simulink model "CML_Iso_Force_Matching"  (R2015a)
settings: Solver=ode4  SolverMode=MultiTasking  StartTime=0.0  StopTime=inf  FixedStep=BKIN_STEP_TIME  RelTol=1e-3
StartFcn:
  |  warndlg('Dexterit-E models cannot run under simulation. Please compile your model and run it from within Dexterit-E.');set_param(bdroot,'SimulationCommand','stop')
model workspace (MAT data in the model file):
  BKIN_STEP_TIME = 0.00025
  col_x = 1
  col_y = 2
  VRAD = 3
  COLOR = 4
  TARGET_COL = 2
  BKIN_KINEMATIC_FRAME_SIZE = 400
  E_NO_EVENT = 0
  INIT_DUR = 5
  TP_ITI = 11
  K_JOINT_ASSESSED = 3
  TEXT1 = 5
  TEXT2 = 6
  HEIGHT = 8
  STROKE_WIDTH = 9
  GOAL_F_PCT = 3
  DO_FDBK = 10
  MAX_MOVE_TIME = 9
  MIN_FORCE = 4
  E_TEST_MVC = 1
  E_HOLD_MVC = 3
  E_EOT = 30
  E_FORCE_TRIAL = 11
  E_HOLD_FORCE = 13
  K_BAR_TGT = 4
  K_MVC_TEXT_TGT = 5
  E_INIT_FORCE = 12
  E_SET_MVC = 2
  TRIAL_TYPE = 1
  TEST_ARM = 8
  E_REST_FORCE = 14
  E_INIT_MATCH_FORCE = 15
  E_HOLD_MATCH_FORCE = 16
  TEXT3 = 7
  K_MVC = 6
  E_ACCEPT_MVC = 5
  ACCEPT_MVC = 2
  REJECT_MVC = 3
  K_ARM1_TGT = 1
  K_ARM2_TGT = 2
  E_FATIGUE_TRIAL = 21
  E_INIT_FATIGUE = 22
  E_HOLD_FATIGUE = 23
  HOLD_TIME = 6
  REST_TIME = 7
  E_CHECK_MVC = 4
  E_REJECT_MVC = 6
  K_SUR_TGT = 7
  K_SUR_TEXT_TGT = 8
  TEXT4 = 10
  AUDIO_FDBK_TYPE = 12
libraries: Video x8, simulink x7, slrtlib x7, General x3, KINARM_loads x3, KINARM_IO x2, KINARM_general x2, xpcnilib x1
(part 2 of 2)

== matlab function CML_Iso_Force_Matching/Subsystem1/Trajectory Arm1/calculate robot scaling/MATLAB Function ==
  data: robot_type input; scaling output; exo_scaling input
function scaling = fcn(robot_type, exo_scaling)
%#codegen

scaling = [0, 0];

%0 = EXO, 1 = EP, 2 = NHP
for n=1:2
    if robot_type(n) == 1
        scaling(n) = 0;
    else
        scaling(n) = exo_scaling(n);
    end
end

== matlab function CML_Iso_Force_Matching/Subsystem1/Trajectory Arm1/Create_Trajectory/Virtual_Trajectory/Extract_Position ==
  settings: fimath=|
      | fimath(...
      | 'RoundMode', 'floor',...
      | 'OverflowMode', 'wrap',...
      | 'ProductMode', 'KeepLSB', 'ProductWordLength', 32,...
      | 'SumMode', 'KeepLSB', 'SumWordLength', 32,...
      | 'CastBeforeSum', false)
  data: u input; position output
function position = fcn(u)

position=[0,0];	%initialization
if length(u)==2	%input is assumed to be (x,y) position, global coordinates, (m)		
	position=u;
else			%input is assumed to be a VCODE
	position(1)=u(3);
	position(2)=u(4);
end

== matlab function CML_Iso_Force_Matching/Subsystem1/Trajectory Arm1/Create_Trajectory/Virtual_Trajectory/Extract_Position1 ==
  settings: fimath=|
      | fimath(...
      | 'RoundMode', 'floor',...
      | 'OverflowMode', 'wrap',...
      | 'ProductMode', 'KeepLSB', 'ProductWordLength', 32,...
      | 'SumMode', 'KeepLSB', 'SumWordLength', 32,...
      | 'CastBeforeSum', false)
  data: u input; position output
function position = fcn(u)

position=[0,0];	%initialization
if length(u)==2	%input is assumed to be (x,y) position, global coordinates, (m)		
	position=u;
else			%input is assumed to be a VCODE
	position(1)=u(3);
	position(2)=u(4);
end

== matlab function CML_Iso_Force_Matching/Force_Fdbk_Bar/MakeBar ==
  data: currforce input; VCODES output; mvc input; goalforce input; VCODE input; heightratio output
function [VCODES,heightratio] = fcn(currforce,mvc,goalforce,VCODE)
%#codegen

%calculate the height ratio to scale the inner bar by
heightratio = currforce/(mvc*goalforce/100); %the top of the bar is always the goal force
if heightratio > 1
    heightratio = 1;
elseif heightratio < 0
    heightratio = 0;
end

%duplicate the rectangle shape; VCODE(2,:) will be the inner fill bar,
% VCODE(1,:) will be the outer border
VCODES = [VCODE; VCODE];

%VCODE(1,:) specifies a fill color and no stroke color; we want to make the
%outline have no fill and a white border
VCODES(2,7) = 0; %remove the stroke width on the inner bar
VCODES(2,10) = VCODES(2,10)*.9; %shrink the width of the inner bar to fill the frame
VCODES(1,5) = createcolor(0,0,0); %set the outer frame fill to black
VCODES(1,6) = createcolor(100,100,100); %set the outer frame stroke to white

%the rectangle has dims (10,11,12) = width (x dir), height (y dir), rot
%we want to scale the inner rect height by the heightratio
VCODES(2,11) = VCODES(2,11)*heightratio;
%we need to edit the y position of the inner bar to keep the base fixed at
%the bottom of the outer frame, by subtracting half the height difference
%between the two bars
VCODES(2,4) = VCODES(2,4) - ( VCODES(1,11) - VCODES(2,11) )/2;  


% 
% %we need to add in a line representing the target height.
% VCODES(3,1) = 4; %set this to be a line segment
% 
% framewidth = VCODES(1,10);
% framecenterx = VCODES(1,3);
% framesidex = framecenterx - framewidth/2;
% 
% frameheight = VCODES(1,11);
% framebottom_pos = VCODES(1,4)-(frameheight/2);
% goaloffset = frameheight*(goalforce/100);
% 
% VCODES(3,3) = framesidex;
% VCODES(3,4) = framebottom_pos+goaloffset;
% VCODES(3,10) = framewidth;
% VCODES(3,11) = 0;
% VCODES(3,6) = createcolor(100,0,0);  %set the goal color to be red

end


function color_value = createcolor(red, green, blue)
% CREATE_COLOR Given percentages of red, green and blue creates an RGB color.
% c = CREATE_COLOR(0, 100, 0) creates a pure green
% c = CREATE_COLOR(20, 0, 20) creates a dark magenta.

    red = bound(red);
    green = bound(green);
    blue = bound(blue);
    
    %convert to RGB bytes
    r = uint32(255 * (red / 100));
    g = uint32(255 * (green / 100));
    b = uint32(255 * (blue / 100));
    
    color_value = bitshift(r, 16) + bitshift(g, 8) + b;
    
end


function color = bound(c)
color = c;
if color < 0 || color > 100
    warning 'Valid values are 0-100'
    if color < 0
        color = 0;
    else
        color = 100;
    end
end
end

== matlab function CML_Iso_Force_Matching/Force_Fdbk_Bar/MakeForceText ==
  data: MVC input; CurrForce input; VCODE_mod output; VCODE input; TrialType input
function VCODE_mod  = fcn(MVC, CurrForce, VCODE, TrialType)
%#codegen

%VCODE_mod = VCODE;


%translate the current (avg) MVC to text
force_whole = int32(floor(double(MVC)));
if (force_whole >= 10) %double digit dollar value
    n1d = int32(floor(double(force_whole)/10));
    n2d = force_whole - n1d*10;
    textwhole = [int2char(int32(n1d)) int2char(int32(n2d))];
else %single digit
    textwhole = int2char(int32(force_whole));
end

force_frac = (MVC-double(force_whole))*100;
if (force_frac < 10)
    textfrac = ['0' int2char(int32(force_frac))];
else
    n1 = int32(floor(double(force_frac)/10));
    n2 = round(force_frac - n1*10);
    textfrac = [int2char(int32(n1)) int2char(int32(n2))];
end

%need to translate text into ascii:
textmvc = [double(textwhole) 46 double(textfrac)];


%translate the current exerted force
force_whole = int32(floor(double(CurrForce)));
if (force_whole >= 10) %double digit dollar value
    n1d = int32(floor(double(force_whole)/10));
    n2d = force_whole - n1d*10;
    textwhole = [int2char(int32(n1d)) int2char(int32(n2d))];
else %single digit
    textwhole = int2char(int32(force_whole));
end

force_frac = (CurrForce-double(force_whole))*100;
if (force_frac < 10)
    textfrac = ['0' int2char(int32(force_frac))];
else
    n1 = int32(floor(double(force_frac)/10));
    n2 = round(force_frac - n1*10);
    textfrac = [int2char(int32(n1)) int2char(int32(n2))];
end

textcurrforce = [double(textwhole) 46 double(textfrac)];


textslash = ' / ';
textslash = double(char(textslash));

%always display the full info to the operator
VCODE(1,2) = 3;

textout = [textcurrforce textslash textmvc 0];

VCODE(1,15:min([15+length(textout)-1,64])) = textout(1:min([length(textout),50])); %write out as many the characters as possible into the VCODE
VCODE(1,min([15+length(textout)+1,64])) = 0;  %terminate the string!


%if this is an MVC trial, also show the current force on the subject screen
if TrialType == 1
    
    VCODE_mod = [VCODE; VCODE];
    
    VCODE_mod(2,2) = 2;
    
    textout = [textcurrforce 0];
    
    VCODE_mod(2,15:min([15+length(textout)-1,64])) = textout(1:min([length(textout),50])); %write out as many the characters as possible into the VCODE
    VCODE_mod(2,min([15+length(textout)+1,64])) = 0;  %terminate the string!


else
    
    %we have to keep the matrix size constant, so if we're not showing
    %anything to the subject we will create an empty VCODE
    VCODE_mod = [VCODE; zeros(size(VCODE))];
    
end









function s = int2char(n)

n = mod(n,10); %make sure we only have 1 digit or we will get a weird character!

s = char(n+int32('0')); %// add the character

== stateflow chart CML_Iso_Force_Matching/Subsystem1/Trajectory Arm1/Create_Trajectory/Virtual_Trajectory/VirtualTrajectory ==
  state Initialization/
    virt_pos = reset_pos;
    // this initialization ensures that the virtual position
    // starts off as something reasonable
    traj_status = 0;   // initialize trajectory status
  state main/
    state wait_for_trigger/
      reset_controller = 0;
    state wait_1_ms_b/
      // wait for controller
      // to be reset
    state on_ramp/
      entry: tick = 0;    // initialize the tick counter
      reset_controller = 0;
      final_pos = target_pos;   // set the final position of the trajectory
      start_pos = virt_pos;   // set the start position of the trajectory
      duration = input_duration;   // store the duration of the trajectory
      traj_status = 1;   // indicate an ongoing trajectory
      during:
      on e_clk: tick++;
      // the trajectory velocity will have a bell shaped profile
      trajectory_shape = tick/duration-sin(2*pi*tick/duration)/(2*pi);
      virt_pos[1] = start_pos[1] + (final_pos[1] - start_pos[1]) * trajectory_shape;
      virt_pos[2] = start_pos[2] + (final_pos[2] - start_pos[2]) * trajectory_shape;
    main -> wait_1_ms_b [order 1] : [(robot_enabled == 1) && (traj_status == -1)]/
        | traj_status = 1;
        | virt_pos = reset_pos;
        | reset_controller = 1;
        | // trajectory was halted and
        | //is now being re-started
    wait_for_trigger -> (junction 20) : e_start
    (junction 20) -> wait_for_trigger [order 2]
    wait_1_ms_b -> (junction 20) : after(1, e_clk)
    (junction 20) -> on_ramp [order 1] : [input_duration>0]
    on_ramp -> wait_for_trigger [order 2] : [robot_enabled == 0]/
        | traj_status = -1;
        | // robot disabled
    on_ramp -> wait_for_trigger [order 1] : after(duration, e_clk)/
        | traj_status = 0
        | // trajectory completed
  state wait_1_ms/
    // wait for controller
    // to be reset
  state task_not_running/
    // wait for task_status to change
    // keep updating virt_pos so that the feedback
    // controller output, which is filtered, does not become
    // huge, resulting in a 'bump' if we don't do this.
    traj_status = 0;
    reset_controller = 0;
    during:
    virt_pos = reset_pos;
  (default) -> Initialization
  Initialization -> wait_for_trigger
  wait_1_ms -> wait_for_trigger : after(1, e_clk)
  task_not_running -> wait_1_ms : [task_status > 0]/
      | reset_controller = 1;
      | // task is running again,
      | // so reset position controller
  main -> task_not_running [order 1] : [task_status == 0]/
      | // means that run_status == 0
      | // AND that torque scaling at
      | // end of task is finished
  data: input_duration input double; target_pos input double size=[1 2]; tick local double; duration local double; reset_pos input double size=[1 2]; task_status input double; pi constant double =3.14159265358979; trajectory_shape local double; virt_pos output double size=[1 2]; traj_status output double; robot_enabled input double; start_pos local double size=[1 2]; final_pos local double size=[1 2]; reset_controller output double
  events: e_clk input RISING_EDGE_EVENT; e_start input RISING_EDGE_EVENT

== matlab function CML_Iso_Force_Matching/Subsystem1/Trajectory Arm1/Create_Trajectory/get_arm_info ==
  settings: fimath=|
      | fimath(...
      | 'RoundMode', 'floor',...
      | 'OverflowMode', 'wrap',...
      | 'ProductMode', 'KeepLSB', 'ProductWordLength', 32,...
      | 'SumMode', 'KeepLSB', 'SumWordLength', 32,...
      | 'CastBeforeSum', false)
  data: position output; task_status output; use_dom_hand input; kinarm_data input; run_status input; scaling input; robot_enabled output
function [position, task_status, robot_enabled]  = fcn(use_dom_hand, kinarm_data, run_status, scaling)
%
% get current hand position and robot enabled status
%
% May 2009
%

hpx_index = 23;
hpy_index = 24;
robot_disabled_index = 37;

%determine which arm to apply the load to
dominant_hand=kinarm_data(3,1);						%kinarm_data(3,1) tells which arm is the dominant arm
if use_dom_hand == 1
	feedback_arm = dominant_hand;
else
	feedback_arm = 3 - dominant_hand;
end

hpx = kinarm_data( feedback_arm, hpx_index );
hpy = kinarm_data( feedback_arm, hpy_index );
position = [hpx hpy];

if kinarm_data( feedback_arm, robot_disabled_index ) == 0;
    robot_enabled = 1;
else
    robot_enabled = 0;
end

% if the task has stopped/paused (i.e. run_status == 0) AND the torques outputs
% have scaled down to 0, then set the task_status = 0.
if run_status == 0 && scaling(feedback_arm) == 0
    task_status = 0;
else
    task_status = 1;
end

== matlab function CML_Iso_Force_Matching/Force_Fdbk_Bar/MakeInstructions ==
  data: TrialType input; goal_force input; dofdbk input; VCODE input; VCODE_mod output; instr_state input
function VCODE_mod  = fcn(TrialType, goal_force, dofdbk, VCODE, instr_state)
%#codegen

VCODE_mod = VCODE;

if TrialType == 2 && instr_state == 1 %if test trial and intsructing flex, modify instructions

    textout = [];
    
    if dofdbk == 1
        
        instruct1 = 'Flex your triceps to ';
        instruct2 = '% (fill the bar).';
    else %if dofdbk == 0
        
        instruct1 = 'Flex your triceps to ';
        instruct2 = '%.';
    end
    
    %translate the goal force to text
    force_whole = int32(floor(double(goal_force)));
    if (force_whole >= 10) %double digit dollar value
        n1d = int32(floor(double(force_whole)/10));
        n2d = force_whole - n1d*10;
        textwhole = [int2char(int32(n1d)) int2char(int32(n2d))];
    else %single digit
        textwhole = int2char(int32(force_whole));
    end
    
    force_frac = (goal_force-double(force_whole))*100;
    if (force_frac < 10)
        textfrac = ['0' int2char(int32(force_frac))];
    else
        n1 = int32(floor(double(force_frac)/10));
        n2 = round(force_frac - n1*10);
        textfrac = [int2char(int32(n1)) int2char(int32(n2))];
    end
    
    %need to translate text into ascii:
    if force_frac < 1 %no fractional percentage
        textforce = [double(textwhole)];
    else %some fractional percentage
        textforce = [double(textwhole) 46 double(textfrac)];
    end
    
    textout = [double(instruct1) textforce double(instruct2) 0];
    


    VCODE_mod(1,15:min([15+length(textout)-1,64])) = textout(1:min([length(textout),50])); %write out as many the characters as possible into the VCODE
    VCODE_mod(1,min([15+length(textout)+1,64])) = 0;  %terminate the string!

end






function s = int2char(n)

n = mod(n,10); %make sure we only have 1 digit or we will get a weird character!

s = char(n+int32('0')); %// add the character

== matlab function CML_Iso_Force_Matching/Subsystem1/Trajectory Arm2/Create_Trajectory/Virtual_Trajectory/Extract_Position ==
  settings: fimath=|
      | fimath(...
      | 'RoundMode', 'floor',...
      | 'OverflowMode', 'wrap',...
      | 'ProductMode', 'KeepLSB', 'ProductWordLength', 32,...
      | 'SumMode', 'KeepLSB', 'SumWordLength', 32,...
      | 'CastBeforeSum', false)
  data: u input; position output
function position = fcn(u)

position=[0,0];	%initialization
if length(u)==2	%input is assumed to be (x,y) position, global coordinates, (m)		
	position=u;
else			%input is assumed to be a VCODE
	position(1)=u(3);
	position(2)=u(4);
end

== matlab function CML_Iso_Force_Matching/Subsystem1/Trajectory Arm2/Create_Trajectory/Virtual_Trajectory/Extract_Position1 ==
  settings: fimath=|
      | fimath(...
      | 'RoundMode', 'floor',...
      | 'OverflowMode', 'wrap',...
      | 'ProductMode', 'KeepLSB', 'ProductWordLength', 32,...
      | 'SumMode', 'KeepLSB', 'SumWordLength', 32,...
      | 'CastBeforeSum', false)
  data: u input; position output
function position = fcn(u)

position=[0,0];	%initialization
if length(u)==2	%input is assumed to be (x,y) position, global coordinates, (m)		
	position=u;
else			%input is assumed to be a VCODE
	position(1)=u(3);
	position(2)=u(4);
end

== stateflow chart CML_Iso_Force_Matching/Subsystem1/Trajectory Arm2/Create_Trajectory/Virtual_Trajectory/VirtualTrajectory ==
  state Initialization/
    virt_pos = reset_pos;
    // this initialization ensures that the virtual position
    // starts off as something reasonable
    traj_status = 0;   // initialize trajectory status
  state main/
    state wait_for_trigger/
      reset_controller = 0;
    state wait_1_ms_b/
      // wait for controller
      // to be reset
    state on_ramp/
      entry: tick = 0;    // initialize the tick counter
      reset_controller = 0;
      final_pos = target_pos;   // set the final position of the trajectory
      start_pos = virt_pos;   // set the start position of the trajectory
      duration = input_duration;   // store the duration of the trajectory
      traj_status = 1;   // indicate an ongoing trajectory
      during:
      on e_clk: tick++;
      // the trajectory velocity will have a bell shaped profile
      trajectory_shape = tick/duration-sin(2*pi*tick/duration)/(2*pi);
      virt_pos[1] = start_pos[1] + (final_pos[1] - start_pos[1]) * trajectory_shape;
      virt_pos[2] = start_pos[2] + (final_pos[2] - start_pos[2]) * trajectory_shape;
    main -> wait_1_ms_b [order 1] : [(robot_enabled == 1) && (traj_status == -1)]/
        | traj_status = 1;
        | virt_pos = reset_pos;
        | reset_controller = 1;
        | // trajectory was halted and
        | //is now being re-started
    wait_for_trigger -> (junction 20) : e_start
    (junction 20) -> wait_for_trigger [order 2]
    wait_1_ms_b -> (junction 20) : after(1, e_clk)
    (junction 20) -> on_ramp [order 1] : [input_duration>0]
    on_ramp -> wait_for_trigger [order 2] : [robot_enabled == 0]/
        | traj_status = -1;
        | // robot disabled
    on_ramp -> wait_for_trigger [order 1] : after(duration, e_clk)/
        | traj_status = 0
        | // trajectory completed
  state wait_1_ms/
    // wait for controller
    // to be reset
  state task_not_running/
    // wait for task_status to change
    // keep updating virt_pos so that the feedback
    // controller output, which is filtered, does not become
    // huge, resulting in a 'bump' if we don't do this.
    traj_status = 0;
    reset_controller = 0;
    during:
    virt_pos = reset_pos;
  (default) -> Initialization
  Initialization -> wait_for_trigger
  wait_1_ms -> wait_for_trigger : after(1, e_clk)
  task_not_running -> wait_1_ms : [task_status > 0]/
      | reset_controller = 1;
      | // task is running again,
      | // so reset position controller
  main -> task_not_running [order 1] : [task_status == 0]/
      | // means that run_status == 0
      | // AND that torque scaling at
      | // end of task is finished
  data: input_duration input double; target_pos input double size=[1 2]; tick local double; duration local double; reset_pos input double size=[1 2]; task_status input double; pi constant double =3.14159265358979; trajectory_shape local double; virt_pos output double size=[1 2]; traj_status output double; robot_enabled input double; start_pos local double size=[1 2]; final_pos local double size=[1 2]; reset_controller output double
  events: e_clk input RISING_EDGE_EVENT; e_start input RISING_EDGE_EVENT

== matlab function CML_Iso_Force_Matching/Subsystem1/Trajectory Arm2/Create_Trajectory/get_arm_info ==
  settings: fimath=|
      | fimath(...
      | 'RoundMode', 'floor',...
      | 'OverflowMode', 'wrap',...
      | 'ProductMode', 'KeepLSB', 'ProductWordLength', 32,...
      | 'SumMode', 'KeepLSB', 'SumWordLength', 32,...
      | 'CastBeforeSum', false)
  data: position output; task_status output; use_dom_hand input; kinarm_data input; run_status input; scaling input; robot_enabled output
function [position, task_status, robot_enabled]  = fcn(use_dom_hand, kinarm_data, run_status, scaling)
%
% get current hand position and robot enabled status
%
% May 2009
%

hpx_index = 23;
hpy_index = 24;
robot_disabled_index = 37;

%determine which arm to apply the load to
dominant_hand=kinarm_data(3,1);						%kinarm_data(3,1) tells which arm is the dominant arm
if use_dom_hand == 1
	feedback_arm = dominant_hand;
else
	feedback_arm = 3 - dominant_hand;
end

hpx = kinarm_data( feedback_arm, hpx_index );
hpy = kinarm_data( feedback_arm, hpy_index );
position = [hpx hpy];

if kinarm_data( feedback_arm, robot_disabled_index ) == 0;
    robot_enabled = 1;
else
    robot_enabled = 0;
end

% if the task has stopped/paused (i.e. run_status == 0) AND the torques outputs
% have scaled down to 0, then set the task_status = 0.
if run_status == 0 && scaling(feedback_arm) == 0
    task_status = 0;
else
    task_status = 1;
end

== matlab function CML_Iso_Force_Matching/Subsystem1/Trajectory Arm2/calculate robot scaling/MATLAB Function ==
  data: robot_type input; scaling output; exo_scaling input
function scaling = fcn(robot_type, exo_scaling)
%#codegen

scaling = [0, 0];

%0 = EXO, 1 = EP, 2 = NHP
for n=1:2
    if robot_type(n) == 1
        scaling(n) = 0;
    else
        scaling(n) = exo_scaling(n);
    end
end

== matlab function CML_Iso_Force_Matching/Play Sound/Play sound over and over ==
  data: tone input; output output; beep input; errorbeep input; coin input; neutral input
function output = fcn(tone,beep,errorbeep,coin,neutral)
%#codegen

persistent t last_tone_state
if isempty(t), t = 0; end
if isempty(last_tone_state), last_tone_state = 0; end

trigger = last_tone_state ~= tone;
if trigger > 0
    last_tone_state = tone;
end

output = 0;		% default
if t == 0 && trigger > 0
	% start the playing of the sound.
	t = t + 1;
end

if neutral==0
    if tone == 1
        data = beep;
    elseif tone == 2
        data = coin;
    elseif tone == 3
        data = errorbeep;
    else 
        t = 0;
        data = 0;
    end
else
    if t>0
        data=beep;
    else
        t=0;
        data=0;
    end
end

if t > 0
	output = data(t);
	if t == length(data)
		t = 0;
	else
		t = t + 1;
	end
end

== matlab function CML_Iso_Force_Matching/Force_Fdbk_Bar/MakeSurveyBar ==
  data: survey_resp input; VCODES output; VCODE input
function VCODES  = fcn(survey_resp,VCODE)
%#codegen

%calculate the height ratio to scale the inner bar by
widthtratio = (survey_resp/8); %the top of the bar is always the max response
if widthtratio > 1
    widthtratio = 1;
elseif widthtratio < 0
    widthtratio = 0;
end


%duplicate the rectangle shape; VCODE(2,:) will be the inner fill bar,
% VCODE(1,:) will be the outer border
VCODES = [VCODE; VCODE];

%VCODE(1,:) specifies a fill color and no stroke color; we want to make the
%outline have no fill and a white border
VCODES(2,7) = 0; %remove the stroke width on the inner bar
VCODES(2,11) = VCODES(2,11)*.9; %shrink the HEIGHT of the inner bar to fill the frame
VCODES(1,5) = createcolor(0,0,0); %set the outer frame fill to black
VCODES(1,6) = createcolor(100,100,100); %set the outer frame stroke to white

%the rectangle has dims (10,11,12) = width (x dir), height (y dir), rot
%we want to scale the inner rect WIDTH by the scale
VCODES(2,10) = VCODES(2,10)*widthtratio;
%we need to edit the y position of the inner bar to keep the base fixed at
%the bottom of the outer frame, by subtracting half the height difference
%between the two bars
VCODES(2,3) = VCODES(2,3) - ( VCODES(1,10) - VCODES(2,10) )/2;  
end

function color_value = createcolor(red, green, blue)
% CREATE_COLOR Given percentages of red, green and blue creates an RGB color.
% c = CREATE_COLOR(0, 100, 0) creates a pure green
% c = CREATE_COLOR(20, 0, 20) creates a dark magenta.

    red = bound(red);
    green = bound(green);
    blue = bound(blue);
    
    %convert to RGB bytes
    r = uint32(255 * (red / 100));
    g = uint32(255 * (green / 100));
    b = uint32(255 * (blue / 100));
    
    color_value = bitshift(r, 16) + bitshift(g, 8) + b;
    
end

function color = bound(c)
color = c;
if color < 0 || color > 100
    warning 'Valid values are 0-100'
    if color < 0
        color = 0;
    else
        color = 100;
    end
end
end

== matlab function CML_Iso_Force_Matching/Force_Fdbk_Bar/MakeSurveyText ==
  data: survey_resp input; TrialType input; VCODE_mod output; VCODE input
function VCODE_mod = fcn(survey_resp,TrialType,VCODE)
% All we're doing here is changing the text to be survey response
% There's a way to  combine them but I dont know it yet
%#codegen

%VCODE_mod = VCODE;

textsurvey = double(int2char(survey_resp));


textslash = ' / ';
textslash = double(char(textslash));
textmax=double(char(' 8 '));

VCODE(1,2) = 3;

textout = [textsurvey textslash textmax];

VCODE(1,15:min([15+length(textout)-1,64])) = textout(1:min([length(textout),50])); %write out as many the characters as possible into the VCODE

VCODE_mod = [VCODE; VCODE];
    
VCODE_mod(2,2) = 2;
    
VCODE_mod(2,15:min([15+length(textout)-1,64])) = textout(1:min([length(textout),50])); %write out as many the characters as possible into the VCODE  %terminate the string!


end

function color_value = createcolor(red, green, blue)
% CREATE_COLOR Given percentages of red, green and blue creates an RGB color.
% c = CREATE_COLOR(0, 100, 0) creates a pure green
% c = CREATE_COLOR(20, 0, 20) creates a dark magenta.

    red = bound(red);
    green = bound(green);
    blue = bound(blue);
    
    %convert to RGB bytes
    r = uint32(255 * (red / 100));
    g = uint32(255 * (green / 100));
    b = uint32(255 * (blue / 100));
    
    color_value = bitshift(r, 16) + bitshift(g, 8) + b;
    
end

function color = bound(c)
color = c;
if color < 0 || color > 100
    warning 'Valid values are 0-100'
    if color < 0
        color = 0;
    else
        color = 100;
    end
end
end

function s = int2char(n)

n = mod(n,10); %make sure we only have 1 digit or we will get a weird character!

s = char(n+int32('0')); %// add the character
end
